simulink model "model"  (R2022a)
settings: Solver=VariableStepAuto  StartTime=0.0  StopTime=1000  RelTol=1e-3
settings Model: Creator=Z0119174  LastModifiedBy=Z0119174

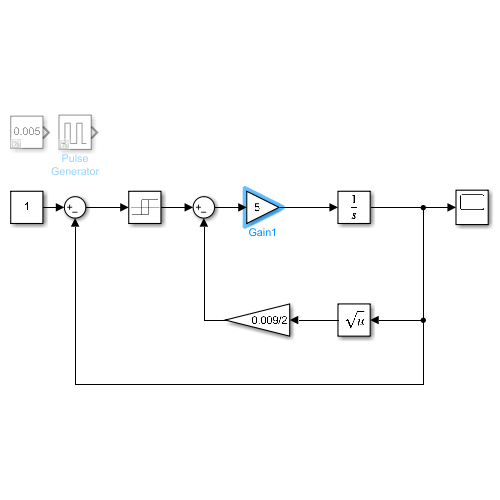
[thumbnail: Simulink's stored preview of the top-level diagram]
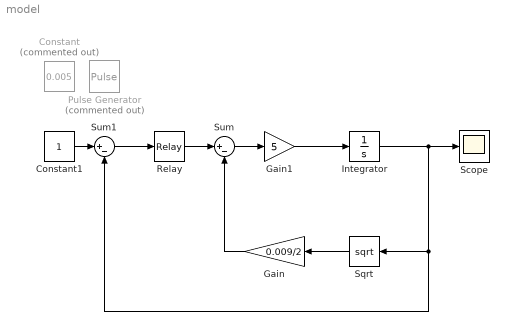
== system model ==
  Constant : Constant  Commented=on  Value=0.005
  Constant1 : Constant
  Gain : Gain  Gain=0.009/2
  Gain1 : Gain  Gain=5
  Integrator : Integrator
  Pulse Generator : DiscretePulseGenerator  Commented=on  PulseType=Time based  Amplitude=0.005  Period=10  PulseWidth=5
  Relay : Relay  OnSwitchValue=0.05  OffSwitchValue=-0.05  OnOutputValue=0.005
  Scope : Scope
  Sqrt : Sqrt
  Sum : Sum  Inputs=|+-
  Sum1 : Sum  Inputs=|+-
  wires:
  Sqrt/1 -> Gain/1
  Relay/1 -> Sum/1
  Gain/1 -> Sum/2
  Sum/1 -> Gain1/1
  Gain1/1 -> Integrator/1
  Sum1/1 -> Relay/1
  Integrator/1 -> Scope/1, Sum1/2, Sqrt/1
  Constant1/1 -> Sum1/1
